simulink model "comm_test_server_vehicle"  (R2014a)
settings: Solver=ode4  StartTime=0.0  StopTime=inf  FixedStep=0.01  RelTol=1e-3
libraries: SimulinkExecutionControl x1
settings Model: Creator=Tulga Ersal  LastModifiedBy=zhengys
settings OptimizationCC: ExpressionDepthLimit=2147483647
settings DebuggingCC: UnderspecifiedInitializationDetection=Classic  StateNameClashWarn=warning

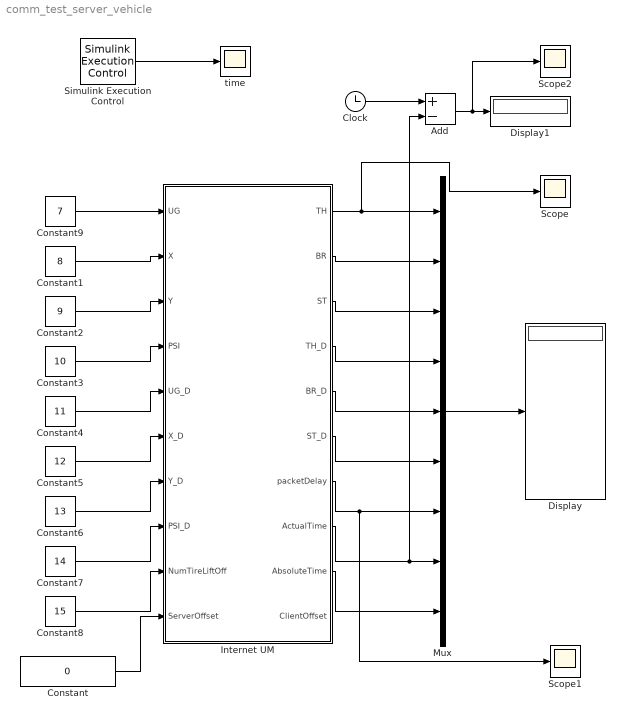
== system comm_test_server_vehicle ==
  Add : Sum  Inputs=+-
  Clock : Clock
  Constant : Constant  Value=0
  Constant1 : Constant  Value=8
  Constant2 : Constant  Value=9
  Constant3 : Constant  Value=10
  Constant4 : Constant  Value=11
  Constant5 : Constant  Value=12
  Constant6 : Constant  Value=13
  Constant7 : Constant  Value=14
  Constant8 : Constant  Value=15
  Constant9 : Constant  Value=7
  Display : Display
  Display1 : Display
  Internet UM : Subsystem
  Mux : Mux  Inputs=9
  Scope : Scope
  Scope1 : Scope
  Scope2 : Scope
      settings: YMin=-0.12  YMax=0.05  SaveName=ScopeData2
  Simulink Execution Control : SimulinkExecutionControl/Simulink Execution Control  proc_pri=REALTIME_PRIORITY_CLASS  thread_pri=THREAD_PRIORITY_TIME_CRITICAL  rt_sim=on  factor=1  ovrrun=Continue execution  Ts=-1
  time : Scope
      settings: TickLabels=on  YMin=1.375  YMax=1.4075  SaveName=ScopeData4
  wires:
  Mux/1 -> Display/1
  Internet UM/5(BR_D) -> Mux/5
  Internet UM/4(TH_D) -> Mux/4
  Internet UM/6(ST_D) -> Mux/6
  Internet UM/3(ST) -> Mux/3
  Internet UM/2(BR) -> Mux/2
  Internet UM/8(ActualTime) -> Mux/8, Add/2
  Internet UM/1(TH) -> Scope/1, Mux/1
  Clock/1 -> Add/1
  Add/1 -> Scope2/1, Display1/1
  Constant9/1 -> Internet UM/1(UG)
  Constant1/1 -> Internet UM/2(X)
  Constant2/1 -> Internet UM/3(Y)
  Constant3/1 -> Internet UM/4(PSI)
  Constant4/1 -> Internet UM/5(UG_D)
  Constant5/1 -> Internet UM/6(X_D)
  Constant6/1 -> Internet UM/7(Y_D)
  Constant7/1 -> Internet UM/8(PSI_D)
  Constant8/1 -> Internet UM/9(NumTireLiftOff)
  Internet UM/9(AbsoluteTime) -> Mux/9
  Internet UM/7(packetDelay) -> Scope1/1, Mux/7
  Simulink Execution Control/1 -> time/1
  Constant/1 -> Internet UM/10(ServerOffset)

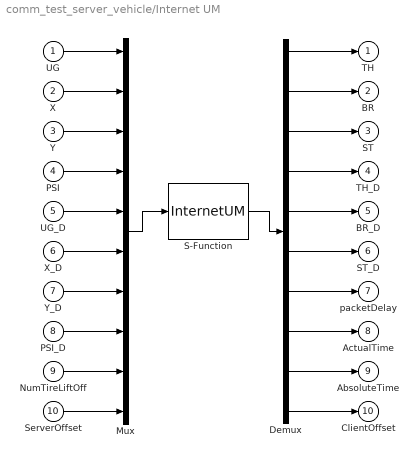
== system comm_test_server_vehicle/Internet UM ==
  UG : Inport
  X : Inport  Port=2
  Y : Inport  Port=3
  PSI : Inport  Port=4
  UG_D : Inport  Port=5
  X_D : Inport  Port=6
  Y_D : Inport  Port=7
  PSI_D : Inport  Port=8
  NumTireLiftOff : Inport  Port=9
  ServerOffset : Inport  Port=10
  Demux : Demux  Outputs=10
  Mux : Mux  Inputs=10
  S-Function : S-Function  FunctionName=InternetUM  EnableBusSupport=off
  TH : Outport
  BR : Outport  Port=2
  ST : Outport  Port=3
  TH_D : Outport  Port=4
  BR_D : Outport  Port=5
  ST_D : Outport  Port=6
  packetDelay : Outport  Port=7
  ActualTime : Outport  Port=8
  AbsoluteTime : Outport  Port=9
  ClientOffset : Outport  Port=10
  wires:
  Mux/1 -> S-Function/1
  S-Function/1 -> Demux/1
  PSI_D/1 -> Mux/8
  Y_D/1 -> Mux/7
  X_D/1 -> Mux/6
  UG_D/1 -> Mux/5
  PSI/1 -> Mux/4
  Y/1 -> Mux/3
  X/1 -> Mux/2
  UG/1 -> Mux/1
  NumTireLiftOff/1 -> Mux/9
  Demux/1 -> TH/1
  Demux/2 -> BR/1
  Demux/3 -> ST/1
  Demux/4 -> TH_D/1
  Demux/5 -> BR_D/1
  Demux/6 -> ST_D/1
  Demux/7 -> packetDelay/1
  Demux/8 -> ActualTime/1
  Demux/9 -> AbsoluteTime/1
  Demux/10 -> ClientOffset/1
  ServerOffset/1 -> Mux/10
